simulink model "simRobotControlSystem_varientGap"  (R2016b)
settings: Solver=VariableStepAuto  StartTime=0.0  StopTime=10.0  RelTol=1e-3
undefined symbols (not defined in the file): Accelerations, Positions, TimeFromStart, Velocities
libraries: robotlib x3
settings Model: Creator=PC15  LastModifiedBy=PC15

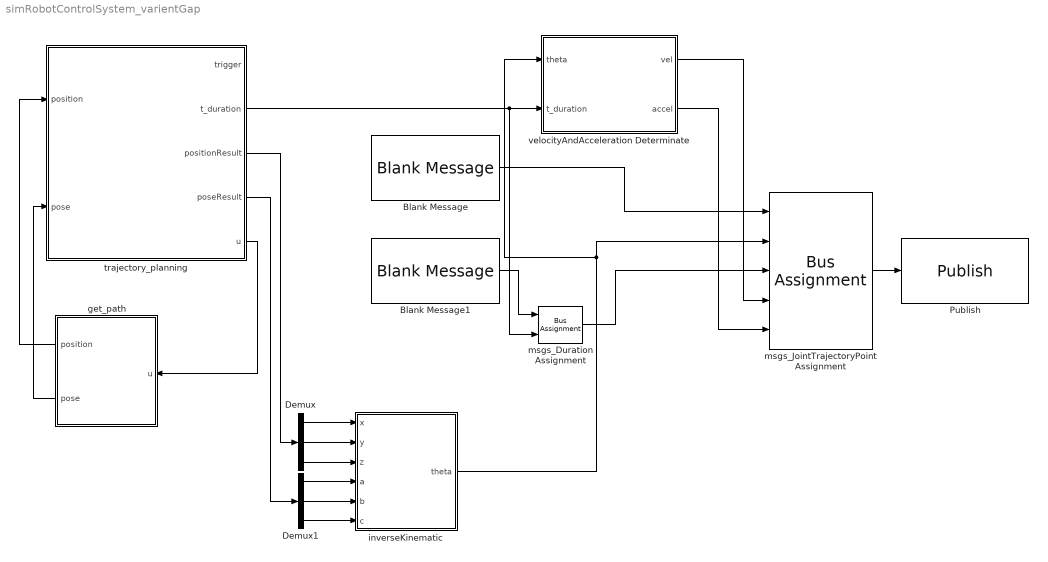
== system simRobotControlSystem_varientGap ==
  Blank Message : robotlib/Blank Message  SourceLibraryInfo=This block requires Robotics System Toolbox  messageType=trajectory_msgs/JointTrajectoryPoint  SampleTime=inf
  Blank Message1 : robotlib/Blank Message  SourceLibraryInfo=This block requires Robotics System Toolbox  messageType=std_msgs/Duration  SampleTime=inf
  Demux : Demux  Outputs=3
  Demux1 : Demux  Outputs=3
  Publish : robotlib/Publish  SourceLibraryInfo=This block requires Robotics System Toolbox  topicSource=Specify your own  topic=/trajectory_topic  messageType=trajectory_msgs/JointTrajectoryPoint  messageQueueLength=1
  get_path : MATLAB Function  TreatAsAtomicUnit=on
  inverseKinematic : MATLAB Function  TreatAsAtomicUnit=on
  msgs_Duration Assignment : BusAssignment  AssignedSignals=Data.Sec
  msgs_JointTrajectoryPoint Assignment : BusAssignment  AssignedSignals=Positions,TimeFromStart,Velocities,Accelerations
  trajectory_planning : MATLAB Function  TreatAsAtomicUnit=on
  velocityAndAcceleration Determinate : MATLAB Function  TreatAsAtomicUnit=on
  wires:
  Blank Message1/1 -> msgs_Duration Assignment/1
  Blank Message/1 -> msgs_JointTrajectoryPoint Assignment/1
  inverseKinematic/1(theta) -> msgs_JointTrajectoryPoint Assignment/2, velocityAndAcceleration Determinate/1(theta)
  msgs_Duration Assignment/1 -> msgs_JointTrajectoryPoint Assignment/3
  msgs_JointTrajectoryPoint Assignment/1 -> Publish/1
  velocityAndAcceleration Determinate/1(vel) -> msgs_JointTrajectoryPoint Assignment/4
  velocityAndAcceleration Determinate/2(accel) -> msgs_JointTrajectoryPoint Assignment/5
  trajectory_planning/5(u) -> get_path/1(u)
  get_path/2(pose) -> trajectory_planning/2(pose)
  get_path/1(position) -> trajectory_planning/1(position)
  trajectory_planning/2(t_duration) -> velocityAndAcceleration Determinate/2(t_duration), msgs_Duration Assignment/2
  trajectory_planning/3(positionResult) -> Demux/1
  Demux1/1 -> inverseKinematic/4(a)
  Demux1/2 -> inverseKinematic/5(b)
  Demux1/3 -> inverseKinematic/6(c)
  Demux/1 -> inverseKinematic/1(x)
  Demux/2 -> inverseKinematic/2(y)
  Demux/3 -> inverseKinematic/3(z)
  trajectory_planning/4(poseResult) -> Demux1/1

== matlab function simRobotControlSystem_varientGap/get_path ==
  data: position output; u input; pose output
function [position,pose] = path_fcn(u)


[x,y,z] = line_function1(u);
[a,b,c] = line_function1(u,'pose');
position=[x;y;z];
pose=[a,b,c];

end

== matlab function simRobotControlSystem_varientGap/inverseKinematic ==
  data: x input; theta output; y input; z input; a input; b input; c input
function theta  = inverseKinematic(x,y,z,a,b,c)

theta = [theta1;theta2;theta3;theta4;theta5;theta6];

== matlab function simRobotControlSystem_varientGap/trajectory_planning ==
  data: trigger output; t_duration output; positionResult output; poseResult output; u output; position input; pose input
function [trigger,t_duration,positionResult,poseResult,u]   = trajectory_planning( position,pose)

t_duration = u;

end

== matlab function simRobotControlSystem_varientGap/velocityAndAcceleration Determinate ==
  data: theta input; vel output; t_duration input; accel output
function [vel,accel] = velAndAccel_calculation(theta,t_duration)

vel=u;
accel=u;
end
